simulink model "scheme1"  (R2024a)
settings: Solver=VariableStepAuto  StartTime=0.0  StopTime=10.0  RelTol=1e-6
values from neighbouring files (symbols this model uses):
  a0 = -2    [main.m]
  a1 = -1    [main.m]
  a2 = 1    [main.m]
  dy0 = 3    [main.m]
  k0 = -3    [main.m]
  k1 = -3    [main.m]
  y0 = 2    [main.m]
settings Model: Creator=alexivanov  LastModifiedBy=alexivanov

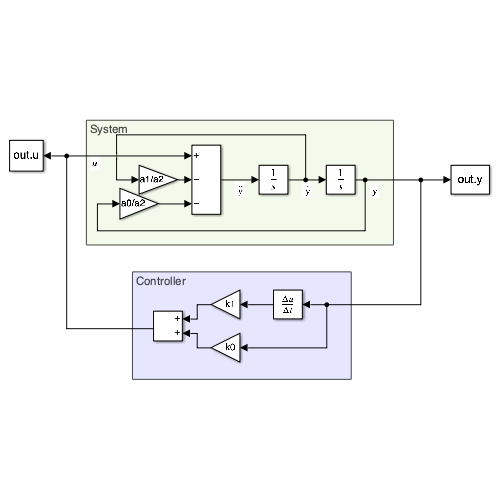
[thumbnail: Simulink's stored preview of the top-level diagram]
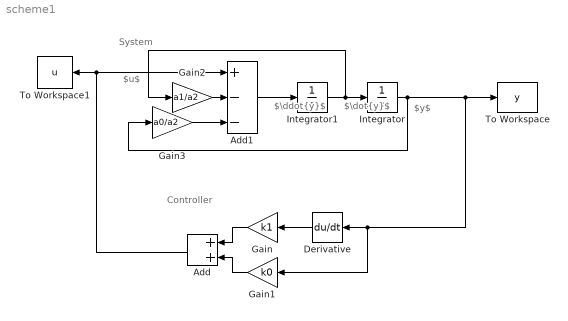
== system scheme1 ==
  note: System
  note: $y$
  note: Controller
  note: $\dot{y}$
  note: $\ddot{y}$
  note: $u$
  Add : Sum
  Add1 : Sum  Inputs=+--
  Derivative : Derivative
  Gain : Gain  Gain=k1
  Gain1 : Gain  Gain=k0
  Gain2 : Gain  Gain=a1/a2
  Gain3 : Gain  Gain=a0/a2
  Integrator : Integrator  InitialCondition=y0
  Integrator1 : Integrator  InitialCondition=dy0
  To Workspace : ToWorkspace  VariableName=y  SaveFormat=Timeseries  SampleTime=-1
  To Workspace1 : ToWorkspace  VariableName=u  SaveFormat=Timeseries  SampleTime=-1
  wires:
  Integrator/1 -> Gain3/1, To Workspace/1, Derivative/1, Gain1/1
  Derivative/1 -> Gain/1
  Gain/1 -> Add/1
  Gain1/1 -> Add/2
  Integrator1/1 -> Gain2/1, Integrator/1
  Add1/1 -> Integrator1/1
  Add/1 -> Add1/1, To Workspace1/1
  Gain2/1 -> Add1/2
  Gain3/1 -> Add1/3
